simulink model "ex02_trafficB"  (R2020b)
settings: Solver=VariableStepAuto  StartTime=0.0  StopTime=60  RelTol=1e-3
model workspace (MAT data in the model file):
  courseObject.course = 'stateflow'
  courseObject.chapter = 3
  courseObject.lesson = 3
  courseObject.section = 1
  courseObject.task = 1
undefined symbols (not defined in the file): sigbuilder_block
settings Model: EnablePacing=on  PacingRate=3  Creator=gb  LastModifiedBy=19255551
settings DataIOCC: SaveTime=off

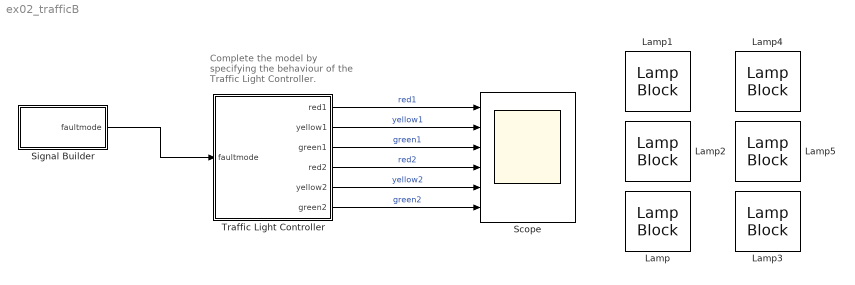
== system ex02_trafficB ==
  note: Complete the model by specifying the behaviour of the Traffic Light Controller.
  Lamp{,1..5} (6 alike) : LampBlock
  Scope : Scope  NumInputPorts=6
  Signal Builder : Subsystem  Tag=STV Subsys  LoadFcn=sigbuilder_block('load');  StartFcn=sigbuilder_block('start');  StopFcn=sigbuilder_block('stop');  ClipboardFcn=sigbuilder_block('clipboard');  mask(Sigbuilder block){tuvar=[0:10]}
      mask help: Simulink:masks:SigbuilderBlock_MD
      mask init:
      | if ~strcmp(get_param(bdroot(gcbh),'SimulationStatus'),'stopped') tuvar = sigbuilder_block('maskInit'); end
      settings: CopyFcn=sigbuilder_block('copy');  DeleteFcn=sigbuilder_block('delete');  ModelCloseFcn=sigbuilder_block('modelClose');  PreSaveFcn=sigbuilder_block('preSave');  PauseFcn=sigbuilder_block('pause');  ContinueFcn=sigbuilder_block('continue');  NameChangeFcn=sigbuilder_block('namechange');  OpenFcn=sigbuilder_block('open',[4.8 22.8 1142.4 538.8 ]);  CloseFcn=sigbuilder_block('close');
      mask Display: plot(0, 0, 100, 100,[2, 2, 32, 32, 2], [68, 8, 8, 68, 68],[32, 2], [38, 38], [32, 19, 2],[53, 60, 44], [32, 17, 17, 2],[16, 16, 31, 31]);txt = getActiveGroup(gcbh);text(2, 100, txt,'verticalAlignment', 'top');
  Traffic Light Controller : Stateflow chart  TreatAsAtomicUnit=on
  wires:
  Traffic Light Controller/3(green1) -> Scope/3  "green1"
  Traffic Light Controller/1(red1) -> Scope/1  "red1"
  Traffic Light Controller/2(yellow1) -> Scope/2  "yellow1"
  Traffic Light Controller/4(red2) -> Scope/4  "red2"
  Traffic Light Controller/5(yellow2) -> Scope/5  "yellow2"
  Traffic Light Controller/6(green2) -> Scope/6  "green2"
  Signal Builder/1(faultmode) -> Traffic Light Controller/1(faultmode)

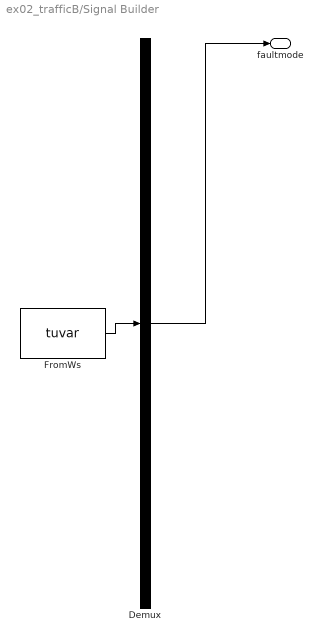
== system ex02_trafficB/Signal Builder ==
  Demux : Demux  Tag=STV Demux  Outputs=1
      settings: DisplayOption=none
  FromWs : FromWorkspace  Tag=STV FromWs  VariableName=tuvar
      SigBuilderData=|
      | common.afterFinalStr = 'Extrapolate'
      | common.sampleTime = 0
      | dataSet.timeRange = [0 60]
      | dataSet.name = 'Group 1'
      | sbobj.Groups.Name = 'Group 1'
      | sbobj.Groups.Signals.Name = 'faultmode'
      | sbobj.Groups.Signals.XData = [0 25 25 40 40 60]
      | sbobj.Groups.Signals.YData = [0 0 1 1 0 0]
      | sbobj.Groups.TimeRange = [0 60]
  faultmode : Outport  Tag=STV Outport
  wires:
  Demux/1 -> faultmode/1
  FromWs/1 -> Demux/1

== stateflow chart ex02_trafficB/Traffic Light Controller ==
  state faultmodeOff
    state Road1Go
      entry:
      green1 = 1;
      red2 = 1;
      red1 = 0;
      yellow2 = 0;
    state Road1Wait
      entry:
      green1 = 0;
      yellow1 = 1;
      red2 = 1;
    state Start
      entry:
      red1 = 1;
      red2 = 1;
      yellow1 = 0;
      yellow2 = 0;
    state Road2Wait
      entry:
      green2 = 0;
      yellow2 = 1;
      red1 = 1;
    state Road2Go
      entry:
      yellow1 = 0;
      red1 = 1;
      green2 = 1;
      red2 = 0;
    (default) -> Start
    Start -> Road1Go : after(5,sec)
    Road1Go -> Road1Wait : after(8,sec)
    Road1Wait -> Road2Go : after(2,sec)
    Road2Wait -> Road1Go : after(2,sec)
    Road2Go -> Road2Wait : after(8,sec)
  state faultmodeOn
    state flashOn
      entry:
      yellow1 = 1;
      yellow2 = 1;
      green1 = 0;
      green2 = 0;
      red1 = 0;
      red2 = 0;
    state flashOff
      entry:
      yellow1 = 0;
      yellow2 = 0;
    (default) -> flashOn
    flashOn -> flashOff : after(1,sec)
    flashOff -> flashOn : after(1,sec)
  (default) -> faultmodeOff
  faultmodeOff -> faultmodeOn : [faultmode == 1]
  faultmodeOn -> faultmodeOff : [faultmode == 0]
  data: red1 output; yellow1 output; green1 output; red2 output; yellow2 output; green2 output; faultmode input
